simulink model "final_test2"  (Simulink 7.7)
settings: Solver=ode45  StartTime=0.0  StopTime=10.0  RelTol=1e-3
undefined symbols (not defined in the file): des_attributefunction_support, des_figposition
libraries: simeventsattributes2 x84, simeventsrouting1 x60, simeventsserver1 x31, commrandsrc2 x24, simeventsgenerators1 x16, simeventstranslate1 x15, simeventssink1 x12, simeventsqueue1 x8
(part 3 of 3)

== system final_test2/Red Link5 ==
  N-Server : simeventsserver1/N-Server  SystemSampleTime=-1  NumberOfServers=2  ServiceTimeFrom=Dialog  ServiceTime=0.001  AttributeName=ServiceTime  PriorityServiceCompletion=500  EnableTOPort=off  StatNumberDeparted=Off  StatNumberInBlock=Off  StatPendingEntity=Off  StatNumberPending=Off  StatAverageWait=Off  StatUtilization=Off  StatNumberTimedout=Off
  Output Switch : simeventsrouting1/Output Switch  SystemSampleTime=-1  NumberOutputPorts=2  SwitchingCriterion=From attribute  InitialSeed=34567  AttributeName=port  InitialConditionsOpt=off  InitialConditions=1  EntityBufferOpt=off  SpecifyEventPriority=off  PriorityOutputSwitchSelectPort=4100  TimeoutPortOpt=off  StatNumberDeparted=Off  StatNumberTimedOut=Off  StatPendingEntity=Off  StatLastDeparturePort=Off  EvaluatedNumPorts=2
  Path Combiner : simeventsrouting1/Path Combiner  SystemSampleTime=-1  NumberInputPorts=2  InputPortPrecedence=IN1 port  InitialSeed=45675  SpecifyEventPriority=off  PriorityPathCombinerPortPrecedenceSelection=4100  StatNumberDeparted=Off  StatLastArrivalPort=Off  EvaluatedNumPorts=2
  Set Attribute : simeventsattributes2/Set Attribute  SystemSampleTime=-1  AttributeFrom=Dialog  AttributeName=port  AttributeTreatAsVector=1  AttributeValue=1  AttributeCreate=on  StatNumberDeparted=Off  EvaluatedAttributeValue={1}
  Set Attribute1 : simeventsattributes2/Set Attribute  SystemSampleTime=-1  AttributeFrom=Dialog  AttributeName=port  AttributeTreatAsVector=1  AttributeValue=2  AttributeCreate=on  StatNumberDeparted=Off  EvaluatedAttributeValue={2}
  Input1 : PMIOPort  Port=1  Side=Left
  Output1 : PMIOPort  Port=2  Side=Right
  Input2 : PMIOPort  Port=3  Side=Right
  Output2 : PMIOPort  Port=4  Side=Left
  connections:
  Set Attribute1/RConn1 -- Path Combiner/LConn2
  Input2/RConn1 -- Set Attribute1/LConn1
  Set Attribute/RConn1 -- Path Combiner/LConn1
  Input1/RConn1 -- Set Attribute/LConn1
  Output Switch/RConn2 -- Output2/RConn1
  Output Switch/RConn1 -- Output1/RConn1
  N-Server/RConn1 -- Output Switch/LConn1
  Path Combiner/RConn1 -- N-Server/LConn1

== system final_test2/Red Link6 ==
  N-Server : simeventsserver1/N-Server  SystemSampleTime=-1  NumberOfServers=2  ServiceTimeFrom=Dialog  ServiceTime=0.001  AttributeName=ServiceTime  PriorityServiceCompletion=500  EnableTOPort=off  StatNumberDeparted=Off  StatNumberInBlock=Off  StatPendingEntity=Off  StatNumberPending=Off  StatAverageWait=Off  StatUtilization=Off  StatNumberTimedout=Off
  Output Switch : simeventsrouting1/Output Switch  SystemSampleTime=-1  NumberOutputPorts=2  SwitchingCriterion=From attribute  InitialSeed=34567  AttributeName=port  InitialConditionsOpt=off  InitialConditions=1  EntityBufferOpt=off  SpecifyEventPriority=off  PriorityOutputSwitchSelectPort=4100  TimeoutPortOpt=off  StatNumberDeparted=Off  StatNumberTimedOut=Off  StatPendingEntity=Off  StatLastDeparturePort=Off  EvaluatedNumPorts=2
  Path Combiner : simeventsrouting1/Path Combiner  SystemSampleTime=-1  NumberInputPorts=2  InputPortPrecedence=IN1 port  InitialSeed=45675  SpecifyEventPriority=off  PriorityPathCombinerPortPrecedenceSelection=4100  StatNumberDeparted=Off  StatLastArrivalPort=Off  EvaluatedNumPorts=2
  Set Attribute : simeventsattributes2/Set Attribute  SystemSampleTime=-1  AttributeFrom=Dialog  AttributeName=port  AttributeTreatAsVector=1  AttributeValue=1  AttributeCreate=on  StatNumberDeparted=Off  EvaluatedAttributeValue={1}
  Set Attribute1 : simeventsattributes2/Set Attribute  SystemSampleTime=-1  AttributeFrom=Dialog  AttributeName=port  AttributeTreatAsVector=1  AttributeValue=2  AttributeCreate=on  StatNumberDeparted=Off  EvaluatedAttributeValue={2}
  Input1 : PMIOPort  Port=1  Side=Left
  Output1 : PMIOPort  Port=2  Side=Right
  Input2 : PMIOPort  Port=3  Side=Right
  Output2 : PMIOPort  Port=4  Side=Left
  connections:
  Path Combiner/RConn1 -- N-Server/LConn1
  N-Server/RConn1 -- Output Switch/LConn1
  Output Switch/RConn1 -- Output1/RConn1
  Output Switch/RConn2 -- Output2/RConn1
  Input1/RConn1 -- Set Attribute/LConn1
  Set Attribute/RConn1 -- Path Combiner/LConn1
  Input2/RConn1 -- Set Attribute1/LConn1
  Set Attribute1/RConn1 -- Path Combiner/LConn2

== system final_test2/Host 1/Attribute Function ==
  Embedded MATLAB Function : Stateflow chart  TreatAsAtomicUnit=on
      settings: PropExecContextOutsideSubsystem=on
  __DEML__EDE2FCE__ : simeventstranslate1/Entity Departure Event to Function-Call Event  Priority=1  SystemSampleTime=-1  TimingFunctionCallF1=Before entity departure  EnableE1Port=off  EnableF2Port=off  TimingFunctionCallF2=Before entity departure  EnableE2Port=off  StatNumberDeparted=Off  StatNumberF1Calls=Off  StatNumberF2Calls=Off  IsInsideAFB=on
  __DEML__GA__ : simeventsattributes2/Get Attribute  Priority=1  SystemSampleTime=-1  AttributeName=type|size  AttributeMissing=Error|Error  AttributeDefaultValue=1|1  AttributeSendTiming=Before entity departure|Before entity departure  AttributeTreatAsVector=1|1  StatNumberDeparted=Off  EvaluatedDefaultAttributeValue={[];[]}
  __DEML__SA__ : simeventsattributes2/Set Attribute  Priority=1  SystemSampleTime=-1  AttributeFrom=Signal port  AttributeName=length  AttributeTreatAsVector=1  AttributeValue=1  AttributeCreate=on  StatNumberDeparted=Off  EvaluatedAttributeValue={[]}
  IN : PMIOPort  Port=1  Side=Left
  OUT : PMIOPort  Port=2  Side=Right
  wires:
  __DEML__EDE2FCE__/1 -> Embedded MATLAB Function/Trigger
  __DEML__GA__/1 -> Embedded MATLAB Function/1(type)
  __DEML__GA__/2 -> Embedded MATLAB Function/2(size)
  Embedded MATLAB Function/1(out_length) -> __DEML__SA__/1
  connections:
  __DEML__SA__/RConn1 -- OUT/RConn1
  IN/RConn1 -- __DEML__GA__/LConn1
  __DEML__GA__/RConn1 -- __DEML__EDE2FCE__/LConn1
  __DEML__EDE2FCE__/RConn1 -- __DEML__SA__/LConn1

== system final_test2/Host 2/Attribute Function ==
  Embedded MATLAB Function : Stateflow chart  TreatAsAtomicUnit=on
      settings: PropExecContextOutsideSubsystem=on
  __DEML__EDE2FCE__ : simeventstranslate1/Entity Departure Event to Function-Call Event  Priority=1  SystemSampleTime=-1  TimingFunctionCallF1=Before entity departure  EnableE1Port=off  EnableF2Port=off  TimingFunctionCallF2=Before entity departure  EnableE2Port=off  StatNumberDeparted=Off  StatNumberF1Calls=Off  StatNumberF2Calls=Off  IsInsideAFB=on
  __DEML__GA__ : simeventsattributes2/Get Attribute  Priority=1  SystemSampleTime=-1  AttributeName=type|size  AttributeMissing=Error|Error  AttributeDefaultValue=1|1  AttributeSendTiming=Before entity departure|Before entity departure  AttributeTreatAsVector=1|1  StatNumberDeparted=Off  EvaluatedDefaultAttributeValue={[];[]}
  __DEML__SA__ : simeventsattributes2/Set Attribute  Priority=1  SystemSampleTime=-1  AttributeFrom=Signal port  AttributeName=length  AttributeTreatAsVector=1  AttributeValue=1  AttributeCreate=on  StatNumberDeparted=Off  EvaluatedAttributeValue={[]}
  IN : PMIOPort  Port=1  Side=Left
  OUT : PMIOPort  Port=2  Side=Right
  wires:
  __DEML__EDE2FCE__/1 -> Embedded MATLAB Function/Trigger
  __DEML__GA__/1 -> Embedded MATLAB Function/1(type)
  __DEML__GA__/2 -> Embedded MATLAB Function/2(size)
  Embedded MATLAB Function/1(out_length) -> __DEML__SA__/1
  connections:
  __DEML__EDE2FCE__/RConn1 -- __DEML__SA__/LConn1
  __DEML__GA__/RConn1 -- __DEML__EDE2FCE__/LConn1
  IN/RConn1 -- __DEML__GA__/LConn1
  __DEML__SA__/RConn1 -- OUT/RConn1

== system final_test2/Host 3/Attribute Function ==
  Embedded MATLAB Function : Stateflow chart  TreatAsAtomicUnit=on
      settings: PropExecContextOutsideSubsystem=on
  __DEML__EDE2FCE__ : simeventstranslate1/Entity Departure Event to Function-Call Event  Priority=1  SystemSampleTime=-1  TimingFunctionCallF1=Before entity departure  EnableE1Port=off  EnableF2Port=off  TimingFunctionCallF2=Before entity departure  EnableE2Port=off  StatNumberDeparted=Off  StatNumberF1Calls=Off  StatNumberF2Calls=Off  IsInsideAFB=on
  __DEML__GA__ : simeventsattributes2/Get Attribute  Priority=1  SystemSampleTime=-1  AttributeName=type|size  AttributeMissing=Error|Error  AttributeDefaultValue=1|1  AttributeSendTiming=Before entity departure|Before entity departure  AttributeTreatAsVector=1|1  StatNumberDeparted=Off  EvaluatedDefaultAttributeValue={[];[]}
  __DEML__SA__ : simeventsattributes2/Set Attribute  Priority=1  SystemSampleTime=-1  AttributeFrom=Signal port  AttributeName=length  AttributeTreatAsVector=1  AttributeValue=1  AttributeCreate=on  StatNumberDeparted=Off  EvaluatedAttributeValue={[]}
  IN : PMIOPort  Port=1  Side=Left
  OUT : PMIOPort  Port=2  Side=Right
  wires:
  __DEML__EDE2FCE__/1 -> Embedded MATLAB Function/Trigger
  __DEML__GA__/1 -> Embedded MATLAB Function/1(type)
  __DEML__GA__/2 -> Embedded MATLAB Function/2(size)
  Embedded MATLAB Function/1(out_length) -> __DEML__SA__/1
  connections:
  __DEML__SA__/RConn1 -- OUT/RConn1
  IN/RConn1 -- __DEML__GA__/LConn1
  __DEML__GA__/RConn1 -- __DEML__EDE2FCE__/LConn1
  __DEML__EDE2FCE__/RConn1 -- __DEML__SA__/LConn1

== system final_test2/Host 4/Attribute Function ==
  Embedded MATLAB Function : Stateflow chart  TreatAsAtomicUnit=on
      settings: PropExecContextOutsideSubsystem=on
  __DEML__EDE2FCE__ : simeventstranslate1/Entity Departure Event to Function-Call Event  Priority=1  SystemSampleTime=-1  TimingFunctionCallF1=Before entity departure  EnableE1Port=off  EnableF2Port=off  TimingFunctionCallF2=Before entity departure  EnableE2Port=off  StatNumberDeparted=Off  StatNumberF1Calls=Off  StatNumberF2Calls=Off  IsInsideAFB=on
  __DEML__GA__ : simeventsattributes2/Get Attribute  Priority=1  SystemSampleTime=-1  AttributeName=type|size  AttributeMissing=Error|Error  AttributeDefaultValue=1|1  AttributeSendTiming=Before entity departure|Before entity departure  AttributeTreatAsVector=1|1  StatNumberDeparted=Off  EvaluatedDefaultAttributeValue={[];[]}
  __DEML__SA__ : simeventsattributes2/Set Attribute  Priority=1  SystemSampleTime=-1  AttributeFrom=Signal port  AttributeName=length  AttributeTreatAsVector=1  AttributeValue=1  AttributeCreate=on  StatNumberDeparted=Off  EvaluatedAttributeValue={[]}
  IN : PMIOPort  Port=1  Side=Left
  OUT : PMIOPort  Port=2  Side=Right
  wires:
  __DEML__EDE2FCE__/1 -> Embedded MATLAB Function/Trigger
  __DEML__GA__/1 -> Embedded MATLAB Function/1(type)
  __DEML__GA__/2 -> Embedded MATLAB Function/2(size)
  Embedded MATLAB Function/1(out_length) -> __DEML__SA__/1
  connections:
  __DEML__EDE2FCE__/RConn1 -- __DEML__SA__/LConn1
  __DEML__GA__/RConn1 -- __DEML__EDE2FCE__/LConn1
  IN/RConn1 -- __DEML__GA__/LConn1
  __DEML__SA__/RConn1 -- OUT/RConn1

== system final_test2/Host 5/Attribute Function ==
  Embedded MATLAB Function : Stateflow chart  TreatAsAtomicUnit=on
      settings: PropExecContextOutsideSubsystem=on
  __DEML__EDE2FCE__ : simeventstranslate1/Entity Departure Event to Function-Call Event  Priority=1  SystemSampleTime=-1  TimingFunctionCallF1=Before entity departure  EnableE1Port=off  EnableF2Port=off  TimingFunctionCallF2=Before entity departure  EnableE2Port=off  StatNumberDeparted=Off  StatNumberF1Calls=Off  StatNumberF2Calls=Off  IsInsideAFB=on
  __DEML__GA__ : simeventsattributes2/Get Attribute  Priority=1  SystemSampleTime=-1  AttributeName=type|size  AttributeMissing=Error|Error  AttributeDefaultValue=1|1  AttributeSendTiming=Before entity departure|Before entity departure  AttributeTreatAsVector=1|1  StatNumberDeparted=Off  EvaluatedDefaultAttributeValue={[];[]}
  __DEML__SA__ : simeventsattributes2/Set Attribute  Priority=1  SystemSampleTime=-1  AttributeFrom=Signal port  AttributeName=length  AttributeTreatAsVector=1  AttributeValue=1  AttributeCreate=on  StatNumberDeparted=Off  EvaluatedAttributeValue={[]}
  IN : PMIOPort  Port=1  Side=Left
  OUT : PMIOPort  Port=2  Side=Right
  wires:
  __DEML__EDE2FCE__/1 -> Embedded MATLAB Function/Trigger
  __DEML__GA__/1 -> Embedded MATLAB Function/1(type)
  __DEML__GA__/2 -> Embedded MATLAB Function/2(size)
  Embedded MATLAB Function/1(out_length) -> __DEML__SA__/1
  connections:
  __DEML__SA__/RConn1 -- OUT/RConn1
  IN/RConn1 -- __DEML__GA__/LConn1
  __DEML__GA__/RConn1 -- __DEML__EDE2FCE__/LConn1
  __DEML__EDE2FCE__/RConn1 -- __DEML__SA__/LConn1

== system final_test2/Host 6/Attribute Function ==
  Embedded MATLAB Function : Stateflow chart  TreatAsAtomicUnit=on
      settings: PropExecContextOutsideSubsystem=on
  __DEML__EDE2FCE__ : simeventstranslate1/Entity Departure Event to Function-Call Event  Priority=1  SystemSampleTime=-1  TimingFunctionCallF1=Before entity departure  EnableE1Port=off  EnableF2Port=off  TimingFunctionCallF2=Before entity departure  EnableE2Port=off  StatNumberDeparted=Off  StatNumberF1Calls=Off  StatNumberF2Calls=Off  IsInsideAFB=on
  __DEML__GA__ : simeventsattributes2/Get Attribute  Priority=1  SystemSampleTime=-1  AttributeName=type|size  AttributeMissing=Error|Error  AttributeDefaultValue=1|1  AttributeSendTiming=Before entity departure|Before entity departure  AttributeTreatAsVector=1|1  StatNumberDeparted=Off  EvaluatedDefaultAttributeValue={[];[]}
  __DEML__SA__ : simeventsattributes2/Set Attribute  Priority=1  SystemSampleTime=-1  AttributeFrom=Signal port  AttributeName=length  AttributeTreatAsVector=1  AttributeValue=1  AttributeCreate=on  StatNumberDeparted=Off  EvaluatedAttributeValue={[]}
  IN : PMIOPort  Port=1  Side=Left
  OUT : PMIOPort  Port=2  Side=Right
  wires:
  __DEML__EDE2FCE__/1 -> Embedded MATLAB Function/Trigger
  __DEML__GA__/1 -> Embedded MATLAB Function/1(type)
  __DEML__GA__/2 -> Embedded MATLAB Function/2(size)
  Embedded MATLAB Function/1(out_length) -> __DEML__SA__/1
  connections:
  __DEML__EDE2FCE__/RConn1 -- __DEML__SA__/LConn1
  __DEML__GA__/RConn1 -- __DEML__EDE2FCE__/LConn1
  IN/RConn1 -- __DEML__GA__/LConn1
  __DEML__SA__/RConn1 -- OUT/RConn1

== system final_test2/Host 7/Attribute Function ==
  Embedded MATLAB Function : Stateflow chart  TreatAsAtomicUnit=on
      settings: PropExecContextOutsideSubsystem=on
  __DEML__EDE2FCE__ : simeventstranslate1/Entity Departure Event to Function-Call Event  Priority=1  SystemSampleTime=-1  TimingFunctionCallF1=Before entity departure  EnableE1Port=off  EnableF2Port=off  TimingFunctionCallF2=Before entity departure  EnableE2Port=off  StatNumberDeparted=Off  StatNumberF1Calls=Off  StatNumberF2Calls=Off  IsInsideAFB=on
  __DEML__GA__ : simeventsattributes2/Get Attribute  Priority=1  SystemSampleTime=-1  AttributeName=type|size  AttributeMissing=Error|Error  AttributeDefaultValue=1|1  AttributeSendTiming=Before entity departure|Before entity departure  AttributeTreatAsVector=1|1  StatNumberDeparted=Off  EvaluatedDefaultAttributeValue={[];[]}
  __DEML__SA__ : simeventsattributes2/Set Attribute  Priority=1  SystemSampleTime=-1  AttributeFrom=Signal port  AttributeName=length  AttributeTreatAsVector=1  AttributeValue=1  AttributeCreate=on  StatNumberDeparted=Off  EvaluatedAttributeValue={[]}
  IN : PMIOPort  Port=1  Side=Left
  OUT : PMIOPort  Port=2  Side=Right
  wires:
  __DEML__EDE2FCE__/1 -> Embedded MATLAB Function/Trigger
  __DEML__GA__/1 -> Embedded MATLAB Function/1(type)
  __DEML__GA__/2 -> Embedded MATLAB Function/2(size)
  Embedded MATLAB Function/1(out_length) -> __DEML__SA__/1
  connections:
  __DEML__SA__/RConn1 -- OUT/RConn1
  IN/RConn1 -- __DEML__GA__/LConn1
  __DEML__GA__/RConn1 -- __DEML__EDE2FCE__/LConn1
  __DEML__EDE2FCE__/RConn1 -- __DEML__SA__/LConn1

== system final_test2/Host 8/Attribute Function ==
  Embedded MATLAB Function : Stateflow chart  TreatAsAtomicUnit=on
      settings: PropExecContextOutsideSubsystem=on
  __DEML__EDE2FCE__ : simeventstranslate1/Entity Departure Event to Function-Call Event  Priority=1  SystemSampleTime=-1  TimingFunctionCallF1=Before entity departure  EnableE1Port=off  EnableF2Port=off  TimingFunctionCallF2=Before entity departure  EnableE2Port=off  StatNumberDeparted=Off  StatNumberF1Calls=Off  StatNumberF2Calls=Off  IsInsideAFB=on
  __DEML__GA__ : simeventsattributes2/Get Attribute  Priority=1  SystemSampleTime=-1  AttributeName=type|size  AttributeMissing=Error|Error  AttributeDefaultValue=1|1  AttributeSendTiming=Before entity departure|Before entity departure  AttributeTreatAsVector=1|1  StatNumberDeparted=Off  EvaluatedDefaultAttributeValue={[];[]}
  __DEML__SA__ : simeventsattributes2/Set Attribute  Priority=1  SystemSampleTime=-1  AttributeFrom=Signal port  AttributeName=length  AttributeTreatAsVector=1  AttributeValue=1  AttributeCreate=on  StatNumberDeparted=Off  EvaluatedAttributeValue={[]}
  IN : PMIOPort  Port=1  Side=Left
  OUT : PMIOPort  Port=2  Side=Right
  wires:
  __DEML__EDE2FCE__/1 -> Embedded MATLAB Function/Trigger
  __DEML__GA__/1 -> Embedded MATLAB Function/1(type)
  __DEML__GA__/2 -> Embedded MATLAB Function/2(size)
  Embedded MATLAB Function/1(out_length) -> __DEML__SA__/1
  connections:
  __DEML__EDE2FCE__/RConn1 -- __DEML__SA__/LConn1
  __DEML__GA__/RConn1 -- __DEML__EDE2FCE__/LConn1
  IN/RConn1 -- __DEML__GA__/LConn1
  __DEML__SA__/RConn1 -- OUT/RConn1

== system final_test2/R1/Attribute Function ==
  Embedded MATLAB Function : Stateflow chart  TreatAsAtomicUnit=on
      settings: PropExecContextOutsideSubsystem=on
  __DEML__EDE2FCE__ : simeventstranslate1/Entity Departure Event to Function-Call Event  Priority=1  SystemSampleTime=-1  TimingFunctionCallF1=Before entity departure  EnableE1Port=off  EnableF2Port=off  TimingFunctionCallF2=Before entity departure  EnableE2Port=off  StatNumberDeparted=Off  StatNumberF1Calls=Off  StatNumberF2Calls=Off  IsInsideAFB=on
  __DEML__GA__ : simeventsattributes2/Get Attribute  Priority=1  SystemSampleTime=-1  AttributeName=dest  AttributeMissing=Error  AttributeDefaultValue=1  AttributeSendTiming=Before entity departure  AttributeTreatAsVector=1  StatNumberDeparted=Off  EvaluatedDefaultAttributeValue={[]}
  __DEML__SA__ : simeventsattributes2/Set Attribute  Priority=1  SystemSampleTime=-1  AttributeFrom=Signal port  AttributeName=port  AttributeTreatAsVector=1  AttributeValue=1  AttributeCreate=on  StatNumberDeparted=Off  EvaluatedAttributeValue={[]}
  IN : PMIOPort  Port=1  Side=Left
  OUT : PMIOPort  Port=2  Side=Right
  wires:
  __DEML__EDE2FCE__/1 -> Embedded MATLAB Function/Trigger
  __DEML__GA__/1 -> Embedded MATLAB Function/1(dest)
  Embedded MATLAB Function/1(out_port) -> __DEML__SA__/1
  connections:
  __DEML__SA__/RConn1 -- OUT/RConn1
  IN/RConn1 -- __DEML__GA__/LConn1
  __DEML__GA__/RConn1 -- __DEML__EDE2FCE__/LConn1
  __DEML__EDE2FCE__/RConn1 -- __DEML__SA__/LConn1

== system final_test2/R2/Attribute Function ==
  Embedded MATLAB Function : Stateflow chart  TreatAsAtomicUnit=on
      settings: PropExecContextOutsideSubsystem=on
  __DEML__EDE2FCE__ : simeventstranslate1/Entity Departure Event to Function-Call Event  Priority=1  SystemSampleTime=-1  TimingFunctionCallF1=Before entity departure  EnableE1Port=off  EnableF2Port=off  TimingFunctionCallF2=Before entity departure  EnableE2Port=off  StatNumberDeparted=Off  StatNumberF1Calls=Off  StatNumberF2Calls=Off  IsInsideAFB=on
  __DEML__GA__ : simeventsattributes2/Get Attribute  Priority=1  SystemSampleTime=-1  AttributeName=rfrom  AttributeMissing=Error  AttributeDefaultValue=1  AttributeSendTiming=Before entity departure  AttributeTreatAsVector=1  StatNumberDeparted=Off  EvaluatedDefaultAttributeValue={[]}
  __DEML__SA__ : simeventsattributes2/Set Attribute  Priority=1  SystemSampleTime=-1  AttributeFrom=Signal port  AttributeName=port  AttributeTreatAsVector=1  AttributeValue=1  AttributeCreate=on  StatNumberDeparted=Off  EvaluatedAttributeValue={[]}
  IN : PMIOPort  Port=1  Side=Left
  OUT : PMIOPort  Port=2  Side=Right
  wires:
  __DEML__EDE2FCE__/1 -> Embedded MATLAB Function/Trigger
  __DEML__GA__/1 -> Embedded MATLAB Function/1(rfrom)
  Embedded MATLAB Function/1(out_port) -> __DEML__SA__/1
  connections:
  __DEML__SA__/RConn1 -- OUT/RConn1
  IN/RConn1 -- __DEML__GA__/LConn1
  __DEML__GA__/RConn1 -- __DEML__EDE2FCE__/LConn1
  __DEML__EDE2FCE__/RConn1 -- __DEML__SA__/LConn1

== system final_test2/R3/Attribute Function ==
  Embedded MATLAB Function : Stateflow chart  TreatAsAtomicUnit=on
      settings: PropExecContextOutsideSubsystem=on
  __DEML__EDE2FCE__ : simeventstranslate1/Entity Departure Event to Function-Call Event  Priority=1  SystemSampleTime=-1  TimingFunctionCallF1=Before entity departure  EnableE1Port=off  EnableF2Port=off  TimingFunctionCallF2=Before entity departure  EnableE2Port=off  StatNumberDeparted=Off  StatNumberF1Calls=Off  StatNumberF2Calls=Off  IsInsideAFB=on
  __DEML__GA__ : simeventsattributes2/Get Attribute  Priority=1  SystemSampleTime=-1  AttributeName=rfrom|dest  AttributeMissing=Error|Error  AttributeDefaultValue=1|1  AttributeSendTiming=Before entity departure|Before entity departure  AttributeTreatAsVector=1|1  StatNumberDeparted=Off  EvaluatedDefaultAttributeValue={[];[]}
  __DEML__SA__ : simeventsattributes2/Set Attribute  Priority=1  SystemSampleTime=-1  AttributeFrom=Signal port  AttributeName=port  AttributeTreatAsVector=1  AttributeValue=1  AttributeCreate=on  StatNumberDeparted=Off  EvaluatedAttributeValue={[]}
  IN : PMIOPort  Port=1  Side=Left
  OUT : PMIOPort  Port=2  Side=Right
  wires:
  __DEML__EDE2FCE__/1 -> Embedded MATLAB Function/Trigger
  __DEML__GA__/1 -> Embedded MATLAB Function/1(rfrom)
  __DEML__GA__/2 -> Embedded MATLAB Function/2(dest)
  Embedded MATLAB Function/1(out_port) -> __DEML__SA__/1
  connections:
  __DEML__SA__/RConn1 -- OUT/RConn1
  IN/RConn1 -- __DEML__GA__/LConn1
  __DEML__GA__/RConn1 -- __DEML__EDE2FCE__/LConn1
  __DEML__EDE2FCE__/RConn1 -- __DEML__SA__/LConn1

== system final_test2/R4/Attribute Function ==
  Embedded MATLAB Function : Stateflow chart  TreatAsAtomicUnit=on
      settings: PropExecContextOutsideSubsystem=on
  __DEML__EDE2FCE__ : simeventstranslate1/Entity Departure Event to Function-Call Event  Priority=1  SystemSampleTime=-1  TimingFunctionCallF1=Before entity departure  EnableE1Port=off  EnableF2Port=off  TimingFunctionCallF2=Before entity departure  EnableE2Port=off  StatNumberDeparted=Off  StatNumberF1Calls=Off  StatNumberF2Calls=Off  IsInsideAFB=on
  __DEML__GA__ : simeventsattributes2/Get Attribute  Priority=1  SystemSampleTime=-1  AttributeName=rfrom|dest  AttributeMissing=Error|Error  AttributeDefaultValue=1|1  AttributeSendTiming=Before entity departure|Before entity departure  AttributeTreatAsVector=1|1  StatNumberDeparted=Off  EvaluatedDefaultAttributeValue={[];[]}
  __DEML__SA__ : simeventsattributes2/Set Attribute  Priority=1  SystemSampleTime=-1  AttributeFrom=Signal port  AttributeName=port  AttributeTreatAsVector=1  AttributeValue=1  AttributeCreate=on  StatNumberDeparted=Off  EvaluatedAttributeValue={[]}
  IN : PMIOPort  Port=1  Side=Left
  OUT : PMIOPort  Port=2  Side=Right
  wires:
  __DEML__EDE2FCE__/1 -> Embedded MATLAB Function/Trigger
  __DEML__GA__/1 -> Embedded MATLAB Function/1(rfrom)
  __DEML__GA__/2 -> Embedded MATLAB Function/2(dest)
  Embedded MATLAB Function/1(out_port) -> __DEML__SA__/1
  connections:
  __DEML__EDE2FCE__/RConn1 -- __DEML__SA__/LConn1
  __DEML__GA__/RConn1 -- __DEML__EDE2FCE__/LConn1
  IN/RConn1 -- __DEML__GA__/LConn1
  __DEML__SA__/RConn1 -- OUT/RConn1

== system final_test2/R5/Attribute Function ==
  Embedded MATLAB Function : Stateflow chart  TreatAsAtomicUnit=on
      settings: PropExecContextOutsideSubsystem=on
  __DEML__EDE2FCE__ : simeventstranslate1/Entity Departure Event to Function-Call Event  Priority=1  SystemSampleTime=-1  TimingFunctionCallF1=Before entity departure  EnableE1Port=off  EnableF2Port=off  TimingFunctionCallF2=Before entity departure  EnableE2Port=off  StatNumberDeparted=Off  StatNumberF1Calls=Off  StatNumberF2Calls=Off  IsInsideAFB=on
  __DEML__GA__ : simeventsattributes2/Get Attribute  Priority=1  SystemSampleTime=-1  AttributeName=rfrom|dest  AttributeMissing=Error|Error  AttributeDefaultValue=1|1  AttributeSendTiming=Before entity departure|Before entity departure  AttributeTreatAsVector=1|1  StatNumberDeparted=Off  EvaluatedDefaultAttributeValue={[];[]}
  __DEML__SA__ : simeventsattributes2/Set Attribute  Priority=1  SystemSampleTime=-1  AttributeFrom=Signal port  AttributeName=port  AttributeTreatAsVector=1  AttributeValue=1  AttributeCreate=on  StatNumberDeparted=Off  EvaluatedAttributeValue={[]}
  IN : PMIOPort  Port=1  Side=Left
  OUT : PMIOPort  Port=2  Side=Right
  wires:
  __DEML__EDE2FCE__/1 -> Embedded MATLAB Function/Trigger
  __DEML__GA__/1 -> Embedded MATLAB Function/1(rfrom)
  __DEML__GA__/2 -> Embedded MATLAB Function/2(dest)
  Embedded MATLAB Function/1(out_port) -> __DEML__SA__/1
  connections:
  __DEML__EDE2FCE__/RConn1 -- __DEML__SA__/LConn1
  __DEML__GA__/RConn1 -- __DEML__EDE2FCE__/LConn1
  IN/RConn1 -- __DEML__GA__/LConn1
  __DEML__SA__/RConn1 -- OUT/RConn1

== system final_test2/R6/Attribute Function ==
  Embedded MATLAB Function : Stateflow chart  TreatAsAtomicUnit=on
      settings: PropExecContextOutsideSubsystem=on
  __DEML__EDE2FCE__ : simeventstranslate1/Entity Departure Event to Function-Call Event  Priority=1  SystemSampleTime=-1  TimingFunctionCallF1=Before entity departure  EnableE1Port=off  EnableF2Port=off  TimingFunctionCallF2=Before entity departure  EnableE2Port=off  StatNumberDeparted=Off  StatNumberF1Calls=Off  StatNumberF2Calls=Off  IsInsideAFB=on
  __DEML__GA__ : simeventsattributes2/Get Attribute  Priority=1  SystemSampleTime=-1  AttributeName=rfrom|dest  AttributeMissing=Error|Error  AttributeDefaultValue=1|1  AttributeSendTiming=Before entity departure|Before entity departure  AttributeTreatAsVector=1|1  StatNumberDeparted=Off  EvaluatedDefaultAttributeValue={[];[]}
  __DEML__SA__ : simeventsattributes2/Set Attribute  Priority=1  SystemSampleTime=-1  AttributeFrom=Signal port  AttributeName=port  AttributeTreatAsVector=1  AttributeValue=1  AttributeCreate=on  StatNumberDeparted=Off  EvaluatedAttributeValue={[]}
  IN : PMIOPort  Port=1  Side=Left
  OUT : PMIOPort  Port=2  Side=Right
  wires:
  __DEML__EDE2FCE__/1 -> Embedded MATLAB Function/Trigger
  __DEML__GA__/1 -> Embedded MATLAB Function/1(rfrom)
  __DEML__GA__/2 -> Embedded MATLAB Function/2(dest)
  Embedded MATLAB Function/1(out_port) -> __DEML__SA__/1
  connections:
  __DEML__SA__/RConn1 -- OUT/RConn1
  IN/RConn1 -- __DEML__GA__/LConn1
  __DEML__GA__/RConn1 -- __DEML__EDE2FCE__/LConn1
  __DEML__EDE2FCE__/RConn1 -- __DEML__SA__/LConn1

== system final_test2/R7/Attribute Function ==
  Embedded MATLAB Function : Stateflow chart  TreatAsAtomicUnit=on
      settings: PropExecContextOutsideSubsystem=on
  __DEML__EDE2FCE__ : simeventstranslate1/Entity Departure Event to Function-Call Event  Priority=1  SystemSampleTime=-1  TimingFunctionCallF1=Before entity departure  EnableE1Port=off  EnableF2Port=off  TimingFunctionCallF2=Before entity departure  EnableE2Port=off  StatNumberDeparted=Off  StatNumberF1Calls=Off  StatNumberF2Calls=Off  IsInsideAFB=on
  __DEML__GA__ : simeventsattributes2/Get Attribute  Priority=1  SystemSampleTime=-1  AttributeName=dest  AttributeMissing=Error  AttributeDefaultValue=1  AttributeSendTiming=Before entity departure  AttributeTreatAsVector=1  StatNumberDeparted=Off  EvaluatedDefaultAttributeValue={[]}
  __DEML__SA__ : simeventsattributes2/Set Attribute  Priority=1  SystemSampleTime=-1  AttributeFrom=Signal port  AttributeName=port  AttributeTreatAsVector=1  AttributeValue=1  AttributeCreate=on  StatNumberDeparted=Off  EvaluatedAttributeValue={[]}
  IN : PMIOPort  Port=1  Side=Left
  OUT : PMIOPort  Port=2  Side=Right
  wires:
  __DEML__EDE2FCE__/1 -> Embedded MATLAB Function/Trigger
  __DEML__GA__/1 -> Embedded MATLAB Function/1(dest)
  Embedded MATLAB Function/1(out_port) -> __DEML__SA__/1
  connections:
  __DEML__EDE2FCE__/RConn1 -- __DEML__SA__/LConn1
  __DEML__GA__/RConn1 -- __DEML__EDE2FCE__/LConn1
  IN/RConn1 -- __DEML__GA__/LConn1
  __DEML__SA__/RConn1 -- OUT/RConn1

== matlab function Host 7/Attribute Function/Embedded MATLAB Function ==
  data: type input double; out_length output double; size input double
  events: trigger input FUNCTION_CALL_EVENT
function out_length  = fcn(type, size)
base = 256;
if (type == 1)
    base = 512;
end
out_length = base * 2^size*8;

== matlab function Host 8/Attribute Function/Embedded MATLAB Function ==
  data: type input double; out_length output double; size input double
  events: trigger input FUNCTION_CALL_EVENT
function out_length  = fcn(type, size)
base = 256;
if (type == 1)
    base = 512;
end
out_length = base * 2^size * 8;

== matlab function R1/Attribute Function/Embedded MATLAB Function ==
  data: out_port output double; dest input double
  events: trigger input FUNCTION_CALL_EVENT
function out_port = fcn(dest)
%FCN    Access and modify attributes with Embedded MATLAB Function 
% 
% Input arguments must match the attribute names.
% Output arguments must be out_<AttributeName>,
% e.g., out_ServiceTime where ServiceTime is the attribute name.
% 
% The output attribute will be created if it is not present.
%
switch dest
    case 0
        out_port = 1;
    case 1
        out_port = 2;
    case 2
        out_port = 3;
    otherwise
        out_port = 4;
end
return

== matlab function R7/Attribute Function/Embedded MATLAB Function ==
  data: dest input double; out_port output double
  events: trigger input FUNCTION_CALL_EVENT
function out_port  = fcn(dest)
%FCN    Access and modify attributes with Embedded MATLAB Function 
% 
% Input arguments must match the attribute names.
% Output arguments must be out_<AttributeName>,
% e.g., out_ServiceTime where ServiceTime is the attribute name.
% 
% The output attribute will be created if it is not present.
%


switch dest
    case 3
        out_port = 1;
    case 4
        out_port = 2;
    case 5
        out_port = 3;
    otherwise
        out_port = 4;
end

return

== matlab function R2/Attribute Function/Embedded MATLAB Function ==
  data: rfrom input double; out_port output double
  events: trigger input FUNCTION_CALL_EVENT
function out_port  = fcn(rfrom)
%FCN    Access and modify attributes with MATLAB 
% 
% Input arguments must match the attribute names.
% Output arguments must be out_<AttributeName>,
% e.g., out_ServiceTime where ServiceTime is the attribute name.
% 
% The output attribute will be created if it is not present.
%
if (rfrom == 1)
    out_port = 2;
else
    out_port = 1;
end

== matlab function R3/Attribute Function/Embedded MATLAB Function ==
  data: rfrom input double; out_port output double; dest input double
  events: trigger input FUNCTION_CALL_EVENT
function out_port  = fcn(rfrom, dest)
%FCN    Access and modify attributes with MATLAB 
% 
% Input arguments must match the attribute names.
% Output arguments must be out_<AttributeName>,
% e.g., out_ServiceTime where ServiceTime is the attribute name.
% 
% The output attribute will be created if it is not present.
%

R2 = 1;
R4 = 2;
R5 = 3;

switch rfrom
    case 2
        out_port = R4;
    case 4
        out_port = R2;
    case 5
        if (dest >= 1 && dest <= 3)
            out_port = R2;
        else
            out_port = R4;
        end
    otherwise
        out_port = R5;
end

== matlab function R4/Attribute Function/Embedded MATLAB Function ==
  data: rfrom input double; out_port output double; dest input double
  events: trigger input FUNCTION_CALL_EVENT
function out_port  = fcn(rfrom, dest)
%FCN    Access and modify attributes with MATLAB 
% 
% Input arguments must match the attribute names.
% Output arguments must be out_<AttributeName>,
% e.g., out_ServiceTime where ServiceTime is the attribute name.
% 
% The output attribute will be created if it is not present.
%

R3 = 1;
R7 = 2;
R6 = 3;

switch rfrom
    case 3
        out_port = R7;
    case 7
        out_port = R3;
    case 6
        if (dest >= 1 && dest <= 3)
            out_port = R3;
        else
            out_port = R7;
        end
    otherwise
        out_port = R6;
end

== matlab function R5/Attribute Function/Embedded MATLAB Function ==
  data: rfrom input double; out_port output double; dest input double
  events: trigger input FUNCTION_CALL_EVENT
function out_port  = fcn(rfrom, dest)
%FCN    Access and modify attributes with MATLAB 
% 
% Input arguments must match the attribute names.
% Output arguments must be out_<AttributeName>,
% e.g., out_ServiceTime where ServiceTime is the attribute name.
% 
% The output attribute will be created if it is not present.
%

R1 = 1;
R6 = 2;
R3 = 3;

switch rfrom
    case 1
        out_port = R6;
    case 6
        out_port = R1;
    case 3
        if (dest >= 1 && dest <= 3)
            out_port = R1;
        else
            out_port = R6;
        end
    otherwise
        out_port = R3;
end

== matlab function R6/Attribute Function/Embedded MATLAB Function ==
  data: rfrom input double; out_port output double; dest input double
  events: trigger input FUNCTION_CALL_EVENT
function out_port  = fcn(rfrom, dest)
%FCN    Access and modify attributes with MATLAB 
% 
% Input arguments must match the attribute names.
% Output arguments must be out_<AttributeName>,
% e.g., out_ServiceTime where ServiceTime is the attribute name.
% 
% The output attribute will be created if it is not present.
%

R5 = 1;
R7 = 2;
R4 = 3;

switch rfrom
    case 5
        out_port = R7;
    case 7
        out_port = R5;
    case 4
        if (dest >= 1 && dest <= 3)
            out_port = R5;
        else
            out_port = R7;
        end
    otherwise
        out_port = R4;
end

== matlab function Host 1/Attribute Function/Embedded MATLAB Function ==
  data: type input double; out_length output double; size input double
  events: trigger input FUNCTION_CALL_EVENT
function out_length  = fcn(type, size)
base = 256;
if (type == 1)
    base = 512;
end
out_length = base * 2^size*8;

== matlab function Host 2/Attribute Function/Embedded MATLAB Function ==
  data: type input double; out_length output double; size input double
  events: trigger input FUNCTION_CALL_EVENT
function out_length  = fcn(type, size)
base = 256;
if (type == 1)
    base = 512;
end
out_length = base * 2^size * 8;

== matlab function Host 3/Attribute Function/Embedded MATLAB Function ==
  data: type input double; out_length output double; size input double
  events: trigger input FUNCTION_CALL_EVENT
function out_length  = fcn(type, size)
base = 256;
if (type == 1)
    base = 512;
end
out_length = base * 2^size * 8;

== matlab function Host 4/Attribute Function/Embedded MATLAB Function ==
  data: type input double; out_length output double; size input double
  events: trigger input FUNCTION_CALL_EVENT
function out_length  = fcn(type, size)
base = 256;
if (type == 1)
    base = 512;
end
out_length = base * 2^size * 8;

== matlab function Host 5/Attribute Function/Embedded MATLAB Function ==
  data: type input double; out_length output double; size input double
  events: trigger input FUNCTION_CALL_EVENT
function out_length  = fcn(type, size)
base = 256;
if (type == 1)
    base = 512;
end
out_length = base * 2^size * 8;

== matlab function Host 6/Attribute Function/Embedded MATLAB Function ==
  data: type input double; out_length output double; size input double
  events: trigger input FUNCTION_CALL_EVENT
function out_length  = fcn(type, size)
base = 256;
if (type == 1)
    base = 512;
end
out_length = base * 2^size * 8;
